simulink model "InverterGyro"  (R2020a)
settings: Solver=ode23tb  StartTime=0.0  StopTime=10.0  MaxStep=Tc
values from neighbouring files (symbols this model uses):
  cp = 40    [LD9_29rpm38.m]
  CTRPIFF_CLIP_RELEASE = 0.05    [InverterGyro_Init.m]
  emf_fb_p = 0.2*k    (= 0.4)    [LD9_29rpm38.m]
  emf_p = 0.08*k    (= 0.16)    [LD9_29rpm38.m]
  emf_valid = 0.25e3    (= 250)    [LD9_29rpm38.m]
  fcut_u_stack_flt = 161    [InverterGyro_Init.m]
  g0 = fcut_u_stack_flt * Tcontrol_INV    (= 0.0268333333333)    [InverterGyro_Init.m]
  g1 = 1 - g0    (= 0.973166666667)    [InverterGyro_Init.m]
  Ibez = In*sqrt(2)    [LD9_29rpm38.m]
  iq_lim = 1.4    [InverterGyro_Init.m]
  J = J    [plant_data.m]
  kalman_gamma = 1.6    [LD9_29rpm38.m]
  kalman_iq_est = 0    [LD9_29rpm38.m]
  kalman_w = kalman_gamma/k    (= 0.32)    [LD9_29rpm38.m]
  ki_inv_d = 18    [InverterGyro_Init.m]
  ki_inv_q = 18    [InverterGyro_Init.m]
  ki_w = 35    [InverterGyro_Init.m]
  kp_inv_d = 2    [InverterGyro_Init.m]
  kp_inv_q = 2    [InverterGyro_Init.m]
  kp_w = 8    [InverterGyro_Init.m]
  La = 1/3*(Lq+Ld)    (= 0.00188)    [LD9_29rpm38.m]
  Lb = 1/3*(Lq-Ld)    (= 0.00028)    [LD9_29rpm38.m]
  Ld_norm = Ld/Lbez    [LD9_29rpm38.m]
  LFi_0 = LFi_d/10    (= 8e-06)    [InverterGyro_Init.m]
  LFi_d = 80e-6    (= 8e-05)    [InverterGyro_Init.m]
  Ll = 5e-6    (= 5e-06)    [LD9_29rpm38.m]
  Lq_norm = Lq/Lbez    [LD9_29rpm38.m]
  Ls_norm = Ls/Lbez    [LD9_29rpm38.m]
  motorc_m_scale = 2/3*Vdc_nom/Ubez    [LD9_29rpm38.m]
  Omega_bez_motor = we_motor    (= 123.066656217)    [LD9_29rpm38.m]
  Omega_bez_plant = Omega_bez_motor * plant_motor_ratio    (= 123.066656217)    [LD9_29rpm38.m]
  Omega_bez_plant_m = Omega_bez_motor_m * plant_motor_ratio    (= 3.07666640542)    [LD9_29rpm38.m]
  phi = Ubez/Omega_bez_plant    [LD9_29rpm38.m]
  RLFi_0 = RLFi_d/3    (= 0.000334933333333)    [InverterGyro_Init.m]
  RLFi_d = 157*0.08*LFi_d    (= 0.0010048)    [InverterGyro_Init.m]
  Rs = 3.15e-3*n_modules    (= 0.0126)    [LD9_29rpm38.m]
  Rs_norm = Rs/Xbez    [LD9_29rpm38.m]
  settle_time = 0.1    [InverterGyro_Init.m]
  sign_speed = 1    [InverterGyro_Init.m]
  spdobs_emf_o_fact = 0    [LD9_29rpm38.m]
  spdobs_emf_q_fact = 0    [LD9_29rpm38.m]
  Tc = 1e-5    (= 1e-05)    [InverterGyro_Init.m]
  Tcontrol_INV = 1/fPWM_INV/2    (= 0.000166666666667)    [InverterGyro_Init.m]
  Tintcom = 100e-3    (= 0.1)    [InverterGyro_Init.m]
  Tload = 0.75*Tnom    (= 60750)    [LD9_29rpm38.m]
  Tnom = 324e3/n_modules    (= 81000)    [LD9_29rpm38.m]
  tref = 2    [InverterGyro_Init.m]
  Tsamp = Tc    (= 1e-05)    [InverterGyro_Init.m]
  udc_min = 0.85    [InverterGyro_Init.m]
  Vdc_nom = Vdc_ref    (= 720)    [InverterGyro_Init.m]    (also in LD9_29rpm38.m = Vdc_ref)
  Vdc_ref = 720    [InverterGyro_Init.m]
  wref = Omega_sim    [InverterGyro_Init.m]
undefined symbols (not defined in the file or in its folder): magnitude
libraries: powerlib x31, simulink x4, simulink_extras x4, cstblocks x1
(part 1 of 2)
settings Model: SimulationMode=accelerator  Creator=i0007573  LastModifiedBy=dbagn
settings SolverCC: ZeroCrossControl=EnableAll

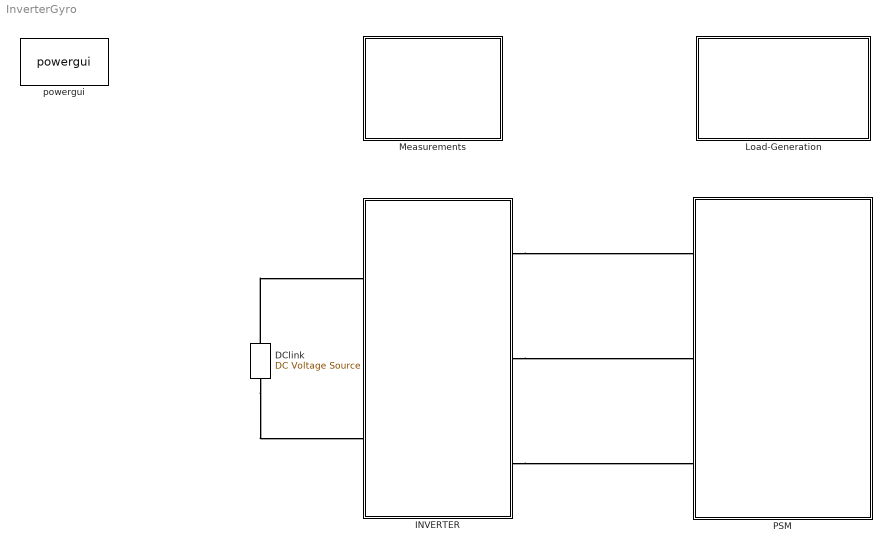
== system InverterGyro ==
  DClink : powerlib/Electrical Sources/DC Voltage Source  Amplitude=Vdc_ref  Measurements=None
  INVERTER : Subsystem
  Load-Generation : Subsystem
  Measurements : Subsystem
  PSM : Subsystem
  powergui : powerlib/powergui  SimulationMode=Continuous  SampleTime=Tc/10  frequency=60  Iterations=50  frequencyindice=0  Pbase=100e6  ErrMax=1e-4  UnitsV=kV  UnitsW=MW  buscounter=0  FunctionMessages=off  echomessages=off  EnableUseOfTLC=off  CurrentSourceSwitches=off  DisableSnubberDevices=off  DisableRonSwitches=off  DisableVfSwitches=off  DisplayEquations=on  AutomaticDiscreteSolvers=off  SolverType=Tustin  Interpol=off  ExternalGateDelay=off  methode=off  Ts=0  x0status=blocks  SPID=off  SwTol=0  HookPort=off  NonlinearTolerance=1e-4  nMaxIteration=100  ContinueOnMaxIteration=off  RestoreLinks=warning  ResistiveCurrentMeasurement=off  Frange=[0:2:500]  Ylog=off  Xlog=on  ShowGrid=off  save=off  variable=ZData  structure=0  ZoomFFT=on  StartTime=0.0  cycles=1  DisplayStyle=1  fundamental=60  FreqAxis=off  MaxFrequency=1000  frequencyindicesteady=1  RmsSteady=1  display=off
  connections:
  INVERTER/RConn1 -- PSM/LConn1
  INVERTER/RConn2 -- PSM/LConn2
  INVERTER/RConn3 -- PSM/LConn3
  DClink/RConn1 -- INVERTER/LConn1
  DClink/LConn1 -- INVERTER/LConn2

== system InverterGyro/INVERTER ==
  GYRO : Subsystem
  INVERTER Control : Subsystem
  LFi4 : powerlib/Elements/Series RLC Branch  LConnTagsString=__new0  RConnTagsString=__new0  BranchType=RL  Resistance=0  Inductance=1e-6  SetiL0=off  InitialCurrent=RLFi  Capacitance=1.0  Setx0=off  InitialVoltage=0  Measurements=Branch voltage and current
  LFi5 : powerlib/Elements/Series RLC Branch  LConnTagsString=__new0  RConnTagsString=__new0  BranchType=RL  Resistance=0  Inductance=1e-6  SetiL0=off  InitialCurrent=RLFi  Capacitance=1.0  Setx0=off  InitialVoltage=0  Measurements=Branch voltage and current
  LFi6 : powerlib/Elements/Series RLC Branch  LConnTagsString=__new0  RConnTagsString=__new0  BranchType=RL  Resistance=0  Inductance=1e-6  SetiL0=off  InitialCurrent=RLFi  Capacitance=1.0  Setx0=off  InitialVoltage=0  Measurements=Branch voltage and current
  LFi_INV1 : powerlib/Elements/Three-Phase Mutual Inductance Z1-Z0  LConnTagsString=a|b|c  RConnTagsString=A|B|C  PositiveSequence=[ RLFi_d LFi_d]  ZeroSequence=[ RLFi_0 LFi_0]
      settings: SourceProductBaseCode=PS
  V1in : PMIOPort  Side=Right
  V2in : PMIOPort  Port=2  Side=Right
  V3in : PMIOPort  Port=3  Side=Right
  DCbus+ : PMIOPort  Port=4  Side=Left
  DCbus- : PMIOPort  Port=5  Side=Left
  wires:
  INVERTER Control/1(PWMout) -> GYRO/1(m)
  connections:
  DCbus-/RConn1 -- GYRO/LConn2
  GYRO/LConn1 -- DCbus+/RConn1
  GYRO/RConn1 -- LFi4/LConn1
  LFi_INV1/RConn1 -- LFi4/RConn1
  LFi_INV1/RConn3 -- LFi6/RConn1
  GYRO/RConn3 -- LFi6/LConn1
  LFi_INV1/RConn2 -- LFi5/RConn1
  GYRO/RConn2 -- LFi5/LConn1
  LFi_INV1/LConn1 -- V1in/RConn1
  LFi_INV1/LConn2 -- V2in/RConn1
  LFi_INV1/LConn3 -- V3in/RConn1

== system InverterGyro/Load-Generation ==
  Gain1 : Gain
  Gain3 : Gain
  Saturation1 : Saturate  UpperLimit=Tload  LowerLimit=0
  To Workspace3 : ToWorkspace  VariableName=Tload_sim  SampleTime=Tc
      settings: MaxDataPoints=Nc
  Transfer Fcn : TransferFcn  Denominator=[1e-2 1]
  tload_ref : simulink/Sources/Ramp  slope=Tnom  start=start_torque_control  InitialOutput=0
  tag scope: Tload_applied=global
  wires:
  tload_ref/1 -> Saturation1/1
  Transfer Fcn/1 -> Gain3/1, To Workspace3/1
  Gain1/1 -> Transfer Fcn/1
  Saturation1/1 -> Gain1/1
  Gain3/1 -> [Tload_applied]

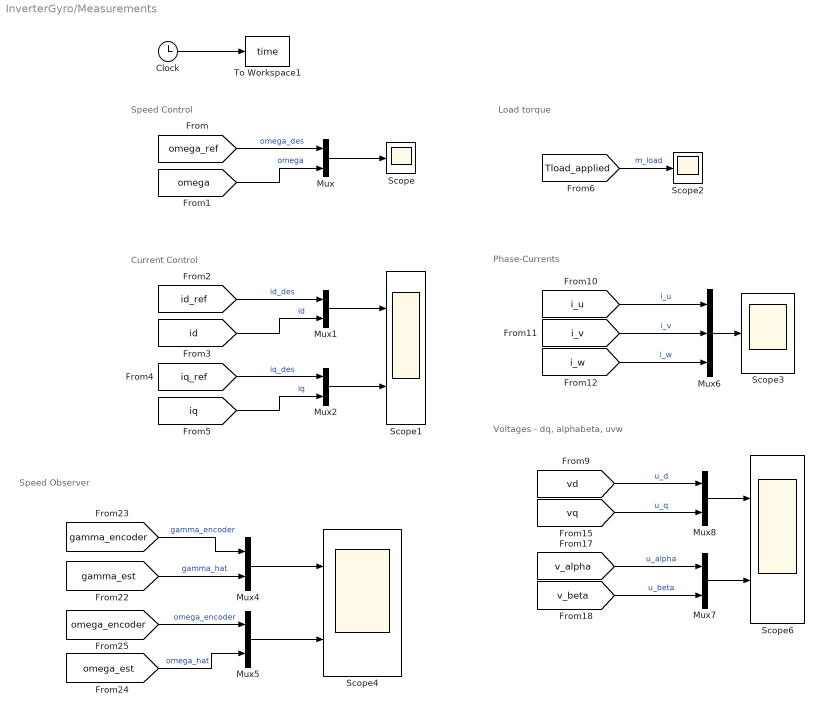
== system InverterGyro/Measurements ==
  note: Speed Observer
  note: Speed Control
  note: Current Control
  note: Load torque
  note: Phase-Currents
  note: Voltages - dq, alphabeta, uvw
  Clock : Clock
  Mux{,1..2,4..5,7..8} (7 alike) : Mux  Inputs=2
  Mux6 : Mux  Inputs=3
  Scope : Scope
  Scope1 : Scope  NumInputPorts=2
  Scope2 : Scope
  Scope3 : Scope
  Scope4 : Scope  NumInputPorts=2
  Scope6 : Scope  NumInputPorts=2
  To Workspace1 : ToWorkspace  VariableName=time  SampleTime=Tc
      settings: MaxDataPoints=Nc
  wires:
  Mux/1 -> Scope/1
  [omega_ref] -> Mux/1  "omega_des"
  [omega] -> Mux/2  "omega"
  Mux1/1 -> Scope1/1
  [id_ref] -> Mux1/1  "id_des"
  [id] -> Mux1/2  "id"
  [iq_ref] -> Mux2/1  "iq_des"
  [iq] -> Mux2/2  "iq"
  Mux2/1 -> Scope1/2
  Mux5/1 -> Scope4/2
  [gamma_encoder] -> Mux4/1  "gamma_encoder"
  Mux4/1 -> Scope4/1
  [omega_encoder] -> Mux5/1  "omega_encoder"
  [omega_est] -> Mux5/2  "omega_hat"
  [gamma_est] -> Mux4/2  "gamma_hat"
  [Tload_applied] -> Scope2/1  "m_load"
  Mux6/1 -> Scope3/1
  [i_u] -> Mux6/1  "i_u"
  [i_v] -> Mux6/2  "i_v"
  [i_w] -> Mux6/3  "i_w"
  [v_beta] -> Mux7/2  "u_beta"
  [v_alpha] -> Mux7/1  "u_alpha"
  [vd] -> Mux8/1  "u_d"
  [vq] -> Mux8/2  "u_q"
  Mux8/1 -> Scope6/1
  Mux7/1 -> Scope6/2
  Clock/1 -> To Workspace1/1

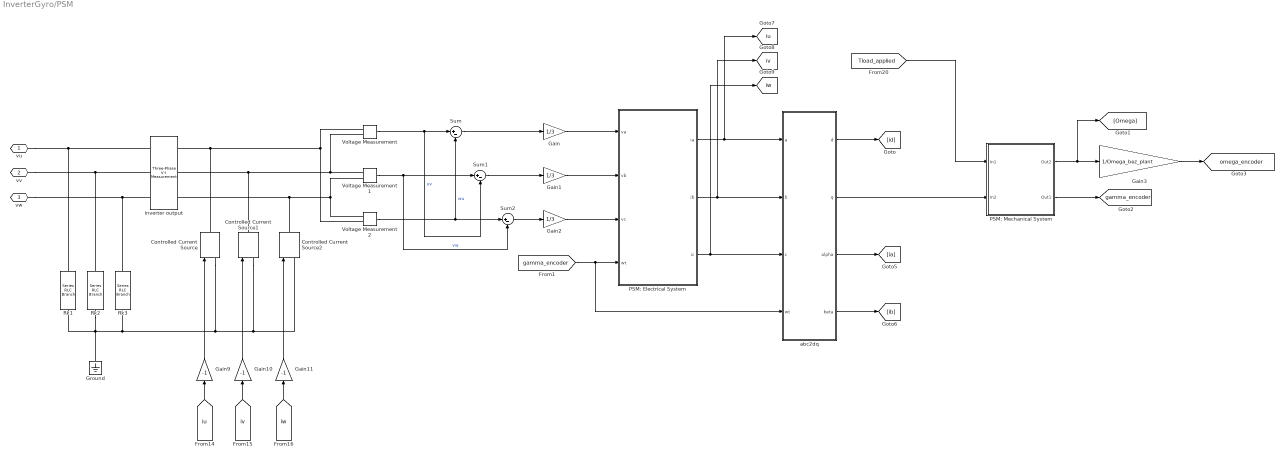
== system InverterGyro/PSM ==
  Controlled Current Source : powerlib/Electrical Sources/Controlled Current Source  Initialize=on  Source_Type=AC  Amplitude=0  Phase=0  Frequency=0  Measurements=None
  Controlled Current Source1 : powerlib/Electrical Sources/Controlled Current Source  Initialize=on  Source_Type=AC  Amplitude=0  Phase=0  Frequency=0  Measurements=None
  Controlled Current Source2 : powerlib/Electrical Sources/Controlled Current Source  Initialize=on  Source_Type=AC  Amplitude=0  Phase=0  Frequency=0  Measurements=None
  Gain : Gain  Gain=1/3
  Gain1 : Gain  Gain=1/3
  Gain10 : Gain  Gain=-1
  Gain11 : Gain  Gain=-1
  Gain2 : Gain  Gain=1/3
  Gain3 : Gain  Gain=1/Omega_bez_plant
  Gain9 : Gain  Gain=-1
  Ground : powerlib/Elements/Ground  LConnTagsString=a
  PSM: Electrical System : Subsystem
  PSM: Mechanical System : Subsystem
  Rk1 : powerlib/Elements/Series RLC Branch  LConnTagsString=__new0  RConnTagsString=__new0  BranchType=R  Resistance=1e6  Inductance=1e-3  SetiL0=off  InitialCurrent=0  Capacitance=1e-6  Setx0=off  InitialVoltage=0  Measurements=Branch voltage
  Rk2 : powerlib/Elements/Series RLC Branch  LConnTagsString=__new0  RConnTagsString=__new0  BranchType=R  Resistance=1e6  Inductance=1e-3  SetiL0=off  InitialCurrent=0  Capacitance=1e-6  Setx0=off  InitialVoltage=0  Measurements=Branch voltage
  Rk3 : powerlib/Elements/Series RLC Branch  LConnTagsString=__new0  RConnTagsString=__new0  BranchType=R  Resistance=1e6  Inductance=1e-3  SetiL0=off  InitialCurrent=0  Capacitance=1e-6  Setx0=off  InitialVoltage=0  Measurements=Branch voltage
  Sum : Sum  Inputs=|+-
  Sum1 : Sum  Inputs=|+-
  Sum2 : Sum  Inputs=|+-
  Voltage Measurement : powerlib/Measurements/Voltage Measurement  PhasorSimulation=off  OutputType=Complex  PSBequivalent=0
  Voltage Measurement1 : powerlib/Measurements/Voltage Measurement  PhasorSimulation=off  OutputType=Complex  PSBequivalent=0
  Voltage Measurement2 : powerlib/Measurements/Voltage Measurement  PhasorSimulation=off  OutputType=Complex  PSBequivalent=0
  "abc2dq " : Subsystem
  inverter output : powerlib/Measurements/Three-Phase V-I Measurement  VoltageMeasurement=phase-to-ground  SetLabelV=on  LabelV=Vgenerator1  Vpu=off  VpuLL=off  CurrentMeasurement=yes  SetLabelI=on  LabelI=Igenerator1  Ipu=off  Pbase=100e6  Vbase=500e3  OutputType=Complex  PhasorSimulation=off  PSBequivalent=0
  vu : PMIOPort  Side=Left
  vv : PMIOPort  Port=2  Side=Left
  vw : PMIOPort  Port=3  Side=Left
  tag scope: gamma_encoder=global, iu=global, iv=global, iw=global, omega_encoder=global
  wires:
  Sum2/1 -> Gain2/1
  Sum1/1 -> Gain1/1
  Sum/1 -> Gain/1
  Voltage Measurement2/1 -> Sum2/1, Sum/2  "wu"
  Voltage Measurement1/1 -> Sum2/2, Sum1/1  "vw"
  Voltage Measurement/1 -> Sum1/2, Sum/1  "uv"
  "abc2dq "/1(d) -> [id]
  [iu] -> Gain9/1
  [iv] -> Gain10/1
  [iw] -> Gain11/1
  Gain9/1 -> Controlled Current Source/1
  Gain10/1 -> Controlled Current Source1/1
  Gain11/1 -> Controlled Current Source2/1
  Gain/1 -> PSM: Electrical System/1(va)
  Gain1/1 -> PSM: Electrical System/2(vb)
  Gain2/1 -> PSM: Electrical System/3(vc)
  PSM: Electrical System/3(ic) -> [iw], "abc2dq "/3(c)
  PSM: Electrical System/2(ib) -> [iv], "abc2dq "/2(b)
  PSM: Electrical System/1(ia) -> [iu], "abc2dq "/1(a)
  "abc2dq "/3(alpha) -> [ia]
  "abc2dq "/4(beta) -> [ib]
  [Tload_applied] -> PSM: Mechanical System/1(In1)
  "abc2dq "/2(q) -> PSM: Mechanical System/2(In2)
  PSM: Mechanical System/1(Out2) -> Gain3/1, [Omega]
  PSM: Mechanical System/2(Out1) -> [gamma_encoder]
  [gamma_encoder] -> "abc2dq "/4(wt), PSM: Electrical System/4(wt)
  Gain3/1 -> [omega_encoder]
  connections:
  Voltage Measurement2/LConn1 -- Controlled Current Source2/RConn1 -- inverter output/RConn1 -- Voltage Measurement1/LConn2
  Voltage Measurement1/LConn1 -- Controlled Current Source1/RConn1 -- inverter output/RConn2 -- Voltage Measurement/LConn2
  Voltage Measurement/LConn1 -- Controlled Current Source/RConn1 -- inverter output/RConn3 -- Voltage Measurement2/LConn2
  Rk1/RConn1 -- Rk2/RConn1 -- Ground/LConn1 -- Controlled Current Source/LConn1 -- Controlled Current Source1/LConn1 -- Controlled Current Source2/LConn1 -- Rk3/RConn1
  Rk3/LConn1 -- vw/RConn1 -- inverter output/LConn1
  Rk2/LConn1 -- vv/RConn1 -- inverter output/LConn2
  Rk1/LConn1 -- vu/RConn1 -- inverter output/LConn3

== system InverterGyro/INVERTER/GYRO ==
  m : Inport
  Demux : Demux  Outputs=3
  Ground : powerlib/Elements/Ground  LConnTagsString=a
  gyro_one_phase : Subsystem
  gyro_one_phase1 : Subsystem
  gyro_one_phase2 : Subsystem
  A : PMIOPort  Side=Right
  B : PMIOPort  Port=2  Side=Right
  C : PMIOPort  Port=3  Side=Right
  V+ : PMIOPort  Port=4  Side=Left
  V- : PMIOPort  Port=5  Side=Left
  wires:
  Demux/1 -> gyro_one_phase/1(m)
  Demux/2 -> gyro_one_phase1/1(m)
  m/1 -> Demux/1
  Demux/3 -> gyro_one_phase2/1(m)
  connections:
  V+/RConn1 -- gyro_one_phase1/LConn1 -- gyro_one_phase2/LConn1 -- gyro_one_phase/LConn1
  V-/RConn1 -- gyro_one_phase/LConn2 -- gyro_one_phase1/LConn2 -- gyro_one_phase2/LConn2
  gyro_one_phase/RConn1 -- A/RConn1
  gyro_one_phase/RConn2 -- gyro_one_phase1/RConn2 -- Ground/LConn1 -- gyro_one_phase2/RConn2
  gyro_one_phase1/RConn1 -- B/RConn1
  gyro_one_phase2/RConn1 -- C/RConn1

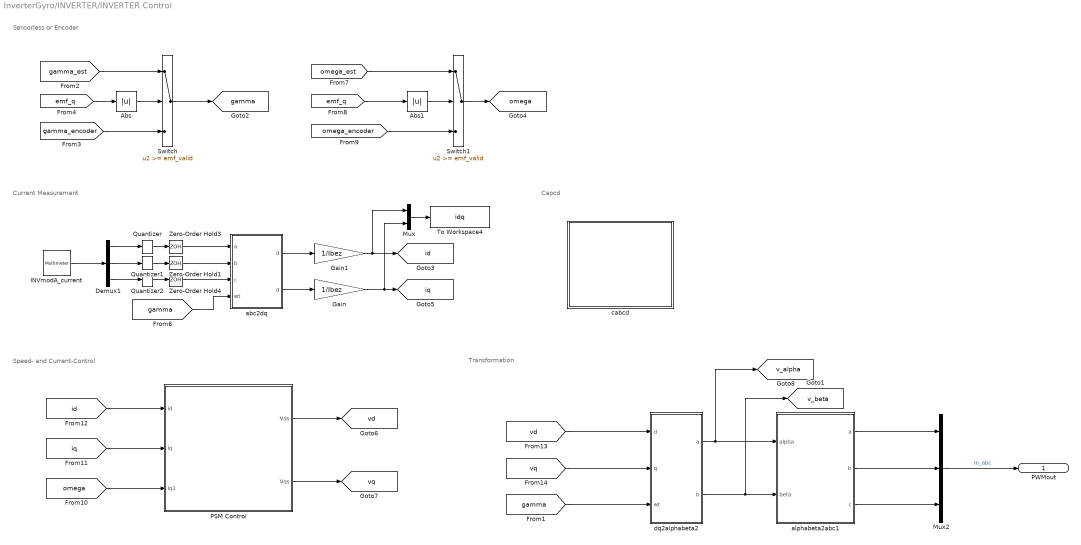
== system InverterGyro/INVERTER/INVERTER Control ==
  note: Capcd
  note: Transformation
  note: Speed- and Current-Control
  note: Current Measurement
  note: Sensorless or Encoder
  Abs : Abs
  Abs1 : Abs
  Demux1 : Demux  Outputs=3
  Gain : Gain  Gain=1/Ibez
  Gain1 : Gain  Gain=1/Ibez
  INVmodA_current : powerlib/Measurements/Multimeter  PhasorSimulation=off  OutputType=Complex  sel=[7 8 9]  L=9  Gain=[1 1 1]  yselected={'Ib: INVERTER/LFi4','Ib: INVERTER/LFi5','Ib: INVERTER/LFi6'};  PSBOutputType=1  PSBequivalent=0  AxesSetting=[0,0.1,-100,100]  Display=0  SavedBlockNames=-11
  Mux : Mux  Inputs=2
  Mux2 : Mux  Inputs=3
  PSM Control : Subsystem
  Quantizer : Quantizer  QuantizationInterval=CurrentQuantization
  Quantizer1 : Quantizer  QuantizationInterval=CurrentQuantization
  Quantizer2 : Quantizer  QuantizationInterval=CurrentQuantization
  Switch : Switch  Threshold=emf_valid
  Switch1 : Switch  Threshold=emf_valid
  To Workspace4 : ToWorkspace  VariableName=idq  SampleTime=Tc
      settings: MaxDataPoints=Nc
  Zero-Order Hold1 : ZeroOrderHold  SampleTime=Tcontrol_INV
  Zero-Order Hold3 : ZeroOrderHold  SampleTime=Tcontrol_INV
  Zero-Order Hold4 : ZeroOrderHold  SampleTime=Tcontrol_INV
  "abc2dq " : Subsystem
  alphabeta2abc1 : Subsystem
  cabcd : Subsystem
  dq2alphabeta2 : Subsystem
  PWMout : Outport
  tag scope: gamma=global, id=global, iq=global, omega=global, v_alpha=global, v_beta=global, vd=global, vq=global
  wires:
  Demux1/2 -> Quantizer1/1
  INVmodA_current/1 -> Demux1/1
  Demux1/3 -> Quantizer2/1
  "abc2dq "/1(d) -> Gain1/1
  "abc2dq "/2(q) -> Gain/1
  Zero-Order Hold3/1 -> "abc2dq "/1(a)
  Zero-Order Hold1/1 -> "abc2dq "/2(b)
  Zero-Order Hold4/1 -> "abc2dq "/3(c)
  Quantizer/1 -> Zero-Order Hold3/1
  Quantizer1/1 -> Zero-Order Hold1/1
  Quantizer2/1 -> Zero-Order Hold4/1
  [gamma_est] -> Switch/1
  [emf_q] -> Abs/1
  Abs/1 -> Switch/2
  Demux1/1 -> Quantizer/1
  [gamma] -> "abc2dq "/4(wt)
  Abs1/1 -> Switch1/2
  [emf_q] -> Abs1/1
  [omega_est] -> Switch1/1
  [omega_encoder] -> Switch1/3
  [omega] -> PSM Control/3(iq1)
  Gain1/1 -> Mux/1, [id]
  Gain/1 -> Mux/2, [iq]
  Mux/1 -> To Workspace4/1
  [id] -> PSM Control/1(id)
  [iq] -> PSM Control/2(iq)
  PSM Control/1(Vds) -> [vd]
  PSM Control/2(Vqs) -> [vq]
  [vd] -> dq2alphabeta2/1(d)
  [vq] -> dq2alphabeta2/2(q)
  [gamma_encoder] -> Switch/3
  Switch/1 -> [gamma]
  Switch1/1 -> [omega]
  dq2alphabeta2/1(a) -> [v_alpha], alphabeta2abc1/1(alpha)
  dq2alphabeta2/2(b) -> [v_beta], alphabeta2abc1/2(beta)
  alphabeta2abc1/1(a) -> Mux2/1
  alphabeta2abc1/2(b) -> Mux2/2
  alphabeta2abc1/3(c) -> Mux2/3
  Mux2/1 -> PWMout/1  "m_abc"
  [gamma] -> dq2alphabeta2/3(wt)

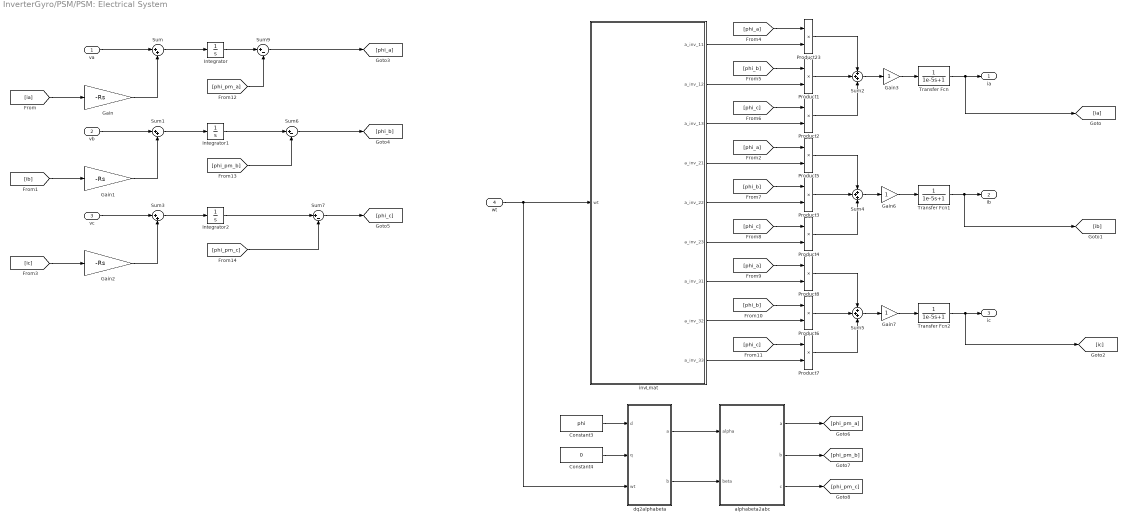
== system InverterGyro/PSM/PSM: Electrical System ==
  va : Inport
  vb : Inport  Port=2
  vc : Inport  Port=3
  wt : Inport  Port=4
  Constant3 : Constant  Value=phi
  Constant4 : Constant  Value=0
  Gain : Gain  Gain=-Rs
  Gain1 : Gain  Gain=-Rs
  Gain2 : Gain  Gain=-Rs
  Gain3 : Gain
  Gain6 : Gain
  Gain7 : Gain
  Integrator : Integrator  InitialCondition=phi
  Integrator1 : Integrator  InitialCondition=phi*cos(2*pi/3)
  Integrator2 : Integrator  InitialCondition=phi*cos(-2*pi/3)
  Product{1..8,23} (9 alike) : Product
  Sum : Sum  Inputs=|++
  Sum1 : Sum  Inputs=|++
  Sum2 : Sum  Inputs=+++
  Sum3 : Sum  Inputs=|++
  Sum4 : Sum  Inputs=+++
  Sum5 : Sum  Inputs=+++
  Sum6 : Sum  Inputs=|+-
  Sum7 : Sum  Inputs=|+-
  Sum9 : Sum  Inputs=|+-
  Transfer Fcn : TransferFcn  Denominator=[1e-5 1]
  Transfer Fcn1 : TransferFcn  Denominator=[1e-5 1]
  Transfer Fcn2 : TransferFcn  Denominator=[1e-5 1]
  alphabeta2abc : Subsystem
  dq2alphabeta : Subsystem
  invLmat : Subsystem
  ia : Outport
  ib : Outport  Port=2
  ic : Outport  Port=3
  wires:
  va/1 -> Sum/1
  Gain/1 -> Sum/2
  [ia] -> Gain/1
  Sum/1 -> Integrator/1
  vb/1 -> Sum1/1
  Gain1/1 -> Sum1/2
  Sum1/1 -> Integrator1/1
  [ib] -> Gain1/1
  vc/1 -> Sum3/1
  Gain2/1 -> Sum3/2
  [ic] -> Gain2/1
  Sum3/1 -> Integrator2/1
  wt/1 -> invLmat/1(wt), dq2alphabeta/3(wt)
  [phi_a] -> Product23/1
  invLmat/1(a_inv_11) -> Product23/2
  [phi_b] -> Product1/1
  invLmat/2(a_inv_12) -> Product1/2
  [phi_c] -> Product2/1
  invLmat/3(a_inv_13) -> Product2/2
  [phi_a] -> Product5/1
  invLmat/4(a_inv_21) -> Product5/2
  [phi_b] -> Product3/1
  invLmat/5(a_inv_22) -> Product3/2
  [phi_c] -> Product4/1
  invLmat/6(a_inv_23) -> Product4/2
  [phi_a] -> Product8/1
  invLmat/7(a_inv_31) -> Product8/2
  [phi_b] -> Product6/1
  invLmat/8(a_inv_32) -> Product6/2
  [phi_c] -> Product7/1
  invLmat/9(a_inv_33) -> Product7/2
  Product1/1 -> Sum2/2
  Product23/1 -> Sum2/1
  Product2/1 -> Sum2/3
  Product3/1 -> Sum4/2
  Product5/1 -> Sum4/1
  Product4/1 -> Sum4/3
  Product6/1 -> Sum5/2
  Product8/1 -> Sum5/1
  Product7/1 -> Sum5/3
  Transfer Fcn2/1 -> [ic], ic/1
  Transfer Fcn1/1 -> [ib], ib/1
  Transfer Fcn/1 -> [ia], ia/1
  Gain7/1 -> Transfer Fcn2/1
  Sum2/1 -> Gain3/1
  Sum4/1 -> Gain6/1
  Sum5/1 -> Gain7/1
  Constant3/1 -> dq2alphabeta/1(d)
  Constant4/1 -> dq2alphabeta/2(q)
  dq2alphabeta/1(a) -> alphabeta2abc/1(alpha)
  dq2alphabeta/2(b) -> alphabeta2abc/2(beta)
  Gain3/1 -> Transfer Fcn/1
  Gain6/1 -> Transfer Fcn1/1
  Integrator/1 -> Sum9/1
  Integrator1/1 -> Sum6/1
  Sum6/1 -> [phi_b]
  Sum7/1 -> [phi_c]
  Integrator2/1 -> Sum7/1
  alphabeta2abc/1(a) -> [phi_pm_a]
  alphabeta2abc/2(b) -> [phi_pm_b]
  alphabeta2abc/3(c) -> [phi_pm_c]
  Sum9/1 -> [phi_a]
  [phi_pm_a] -> Sum9/2
  [phi_pm_b] -> Sum6/2
  [phi_pm_c] -> Sum7/2

== system InverterGyro/PSM/PSM: Mechanical System ==
  In1 : Inport
  In2 : Inport  Port=2
  Constant : Constant  Value=phi
  Constant2 : Constant  Value=2*pi
  Gain5 : Gain  Gain=cp
  Gain6 : Gain  Gain=cp
  Gain8 : Gain  Gain=3/2
  Integrator : Integrator
  Integrator1 : Integrator
  Math Function2 : Math  Operator=mod  SignedPower=on  SaturateOnIntegerOverflow=on
  Product : Product
  Product1 : Product
  Sum5 : Sum  Inputs=|+-
  plant_inertia : Subsystem
  Out2 : Outport
  Out1 : Outport  Port=2
  wires:
  Integrator/1 -> Gain6/1
  Gain6/1 -> Integrator1/1, Out2/1, [Omega]  "Omega"
  plant_inertia/1(J_1) -> Product1/2
  In2/1 -> [iq], Product/1  "iq"
  Integrator1/1 -> Math Function2/1  "wt"
  Constant/1 -> Product/2
  Gain8/1 -> [Te], Sum5/1
  Constant2/1 -> Math Function2/2
  Gain5/1 -> Gain8/1
  Sum5/1 -> Product1/1
  Product/1 -> Gain5/1
  Math Function2/1 -> Out1/1, [theta_m]  "gamma"
  Product1/1 -> Integrator/1
  In1/1 -> Sum5/2  "m_load"

== system InverterGyro/PSM/abc2dq  ==
  a : Inport
  b : Inport  Port=2
  c : Inport  Port=3
  wt : Inport  Port=4
  abc2alphabeta : Subsystem
  alphabeta2dq : Subsystem
  d : Outport
  q : Outport  Port=2
  alpha : Outport  Port=3
  beta : Outport  Port=4
  wires:
  c/1 -> abc2alphabeta/3(c)
  b/1 -> abc2alphabeta/2(b)
  a/1 -> abc2alphabeta/1(a)
  abc2alphabeta/1("alpha ") -> alpha/1, alphabeta2dq/1(alpha)
  abc2alphabeta/2("beta ") -> beta/1, alphabeta2dq/2(beta)
  wt/1 -> alphabeta2dq/3(wt)
  alphabeta2dq/1(d) -> d/1
  alphabeta2dq/2(q) -> q/1

== system InverterGyro/INVERTER/GYRO/gyro_one_phase ==
  m : Inport
  Controlled Current Source2 : powerlib/Electrical Sources/Controlled Current Source  Initialize=on  Source_Type=AC  Amplitude=0  Phase=0  Frequency=0  Measurements=None
  Controlled Voltage Source : powerlib/Electrical Sources/Controlled Voltage Source  Initialize=on  Source_Type=AC  Amplitude=0  Phase=0  Frequency=0  Measurements=None
  Current Measurement : powerlib/Measurements/Current Measurement  PhasorSimulation=off  OutputType=Complex  PSBequivalent=0
  Product : Product
  Product1 : Product
  Transfer Fcn1 : TransferFcn  Denominator=[1e-4 1]
  Transfer Fcn2 : TransferFcn  Denominator=[1e-4 1]
  Voltage Measurement : powerlib/Measurements/Voltage Measurement  PhasorSimulation=off  OutputType=Complex  PSBequivalent=0
  A : PMIOPort  Side=Left
  B : PMIOPort  Port=2  Side=Left
  a : PMIOPort  Port=3  Side=Right
  b : PMIOPort  Port=4  Side=Right
  wires:
  m/1 -> Product1/2, Product/2
  Product/1 -> Controlled Voltage Source/1
  Voltage Measurement/1 -> Transfer Fcn2/1
  Product1/1 -> Controlled Current Source2/1
  Current Measurement/1 -> Transfer Fcn1/1
  Transfer Fcn2/1 -> Product/1
  Transfer Fcn1/1 -> Product1/1
  connections:
  A/RConn1 -- Voltage Measurement/LConn1 -- Controlled Current Source2/LConn1
  Controlled Current Source2/RConn1 -- B/RConn1 -- Voltage Measurement/LConn2
  Controlled Voltage Source/LConn1 -- b/RConn1
  Controlled Voltage Source/RConn1 -- Current Measurement/LConn1
  Current Measurement/RConn1 -- a/RConn1

== system InverterGyro/INVERTER/GYRO/gyro_one_phase1 ==
  m : Inport
  Controlled Current Source2 : powerlib/Electrical Sources/Controlled Current Source  Initialize=on  Source_Type=AC  Amplitude=0  Phase=0  Frequency=0  Measurements=None
  Controlled Voltage Source : powerlib/Electrical Sources/Controlled Voltage Source  Initialize=on  Source_Type=AC  Amplitude=0  Phase=0  Frequency=0  Measurements=None
  Current Measurement : powerlib/Measurements/Current Measurement  PhasorSimulation=off  OutputType=Complex  PSBequivalent=0
  Product : Product
  Product1 : Product
  Transfer Fcn1 : TransferFcn  Denominator=[1e-4 1]
  Transfer Fcn2 : TransferFcn  Denominator=[1e-4 1]
  Voltage Measurement : powerlib/Measurements/Voltage Measurement  PhasorSimulation=off  OutputType=Complex  PSBequivalent=0
  A : PMIOPort  Side=Left
  B : PMIOPort  Port=2  Side=Left
  a : PMIOPort  Port=3  Side=Right
  b : PMIOPort  Port=4  Side=Right
  wires:
  m/1 -> Product1/2, Product/2
  Product/1 -> Controlled Voltage Source/1
  Voltage Measurement/1 -> Transfer Fcn2/1
  Product1/1 -> Controlled Current Source2/1
  Current Measurement/1 -> Transfer Fcn1/1
  Transfer Fcn2/1 -> Product/1
  Transfer Fcn1/1 -> Product1/1
  connections:
  A/RConn1 -- Voltage Measurement/LConn1 -- Controlled Current Source2/LConn1
  Controlled Current Source2/RConn1 -- B/RConn1 -- Voltage Measurement/LConn2
  Controlled Voltage Source/LConn1 -- b/RConn1
  Controlled Voltage Source/RConn1 -- Current Measurement/LConn1
  Current Measurement/RConn1 -- a/RConn1

== system InverterGyro/INVERTER/GYRO/gyro_one_phase2 ==
  m : Inport
  Controlled Current Source2 : powerlib/Electrical Sources/Controlled Current Source  Initialize=on  Source_Type=AC  Amplitude=0  Phase=0  Frequency=0  Measurements=None
  Controlled Voltage Source : powerlib/Electrical Sources/Controlled Voltage Source  Initialize=on  Source_Type=AC  Amplitude=0  Phase=0  Frequency=0  Measurements=None
  Current Measurement : powerlib/Measurements/Current Measurement  PhasorSimulation=off  OutputType=Complex  PSBequivalent=0
  Product : Product
  Product1 : Product
  Transfer Fcn1 : TransferFcn  Denominator=[1e-4 1]
  Transfer Fcn2 : TransferFcn  Denominator=[1e-4 1]
  Voltage Measurement : powerlib/Measurements/Voltage Measurement  PhasorSimulation=off  OutputType=Complex  PSBequivalent=0
  A : PMIOPort  Side=Left
  B : PMIOPort  Port=2  Side=Left
  a : PMIOPort  Port=3  Side=Right
  b : PMIOPort  Port=4  Side=Right
  wires:
  m/1 -> Product1/2, Product/2
  Product/1 -> Controlled Voltage Source/1
  Voltage Measurement/1 -> Transfer Fcn2/1
  Product1/1 -> Controlled Current Source2/1
  Current Measurement/1 -> Transfer Fcn1/1
  Transfer Fcn2/1 -> Product/1
  Transfer Fcn1/1 -> Product1/1
  connections:
  A/RConn1 -- Voltage Measurement/LConn1 -- Controlled Current Source2/LConn1
  Controlled Current Source2/RConn1 -- B/RConn1 -- Voltage Measurement/LConn2
  Controlled Voltage Source/LConn1 -- b/RConn1
  Controlled Voltage Source/RConn1 -- Current Measurement/LConn1
  Current Measurement/RConn1 -- a/RConn1

== system InverterGyro/INVERTER/INVERTER Control/PSM Control ==
  note: EMF & Luenberger Observer
  note: Current Control
  note: Speed Control
  id : Inport
  iq : Inport  Port=2
  iq1 : Inport  Port=3
  Current control : Subsystem
  References : Subsystem
  Speed control : Subsystem
  observer : Subsystem
  speed reference : Subsystem
  Vds : Outport
  Vqs : Outport  Port=2
  tag scope: T_ref=global, gamma_est=global, iq_est=global, omega_est=global
  wires:
  References/1(Id_ref) -> Current control/1(Id_ref)
  References/2(Iq_ref) -> Current control/2(Iq_ref)
  Current control/1(vd) -> Vds/1  "vd"
  Current control/2(vq) -> Vqs/1  "vq"
  speed reference/1(ref_out) -> Speed control/2(Speed ref)
  [i_alpha] -> observer/1(ia_s)
  [i_beta] -> observer/2(ib_s)
  Speed control/1(Torque ref) -> [T_ref]
  [v_alpha] -> observer/3(va_s)
  [v_beta] -> observer/4(vb_s)
  observer/3(iq_hat) -> [iq_est]
  iq1/1 -> Speed control/1(Rotor speed), Current control/3(omega)  "omega"
  id/1 -> Current control/4(id)  "id"
  iq/1 -> Current control/5(iq)  "iq"
  observer/1(iq_hat2) -> [omega_est]
  observer/2(iq_hat1) -> [gamma_est]

== system InverterGyro/INVERTER/INVERTER Control/abc2dq  ==
  a : Inport
  b : Inport  Port=2
  c : Inport  Port=3
  wt : Inport  Port=4
  1/Ti1 : Gain  Gain=1/Ibez  SaturateOnIntegerOverflow=on  OutDataTypeStr=Inherit: Same as input  ParamDataTypeStr=Inherit: Same as input
  1/Ti2 : Gain  Gain=1/Ibez  SaturateOnIntegerOverflow=on  OutDataTypeStr=Inherit: Same as input  ParamDataTypeStr=Inherit: Same as input
  To Workspace1 : ToWorkspace  VariableName=ib  SampleTime=Tc
      settings: MaxDataPoints=Nc
  To Workspace2 : ToWorkspace  VariableName=iq  SampleTime=Tc
      settings: MaxDataPoints=Nc
  To Workspace3 : ToWorkspace  VariableName=id  SampleTime=Tc
      settings: MaxDataPoints=Nc
  To Workspace4 : ToWorkspace  VariableName=ia  SampleTime=Tc
      settings: MaxDataPoints=Nc
  abc2alphabeta : Subsystem
  alphabeta2dq : Subsystem
  d : Outport
  q : Outport  Port=2
  tag scope: i_alpha=global, i_beta=global, i_u=global, i_v=global, i_w=global
  wires:
  wt/1 -> alphabeta2dq/3(wt)  "gamma"
  abc2alphabeta/2("beta ") -> To Workspace1/1, 1/Ti1/1, alphabeta2dq/2(beta)
  abc2alphabeta/1("alpha ") -> 1/Ti2/1, To Workspace4/1, alphabeta2dq/1(alpha)
  a/1 -> [i_u], abc2alphabeta/1(a)
  b/1 -> [i_v], abc2alphabeta/2(b)
  c/1 -> [i_w], abc2alphabeta/3(c)
  1/Ti2/1 -> [i_alpha]
  1/Ti1/1 -> [i_beta]
  alphabeta2dq/2(q) -> To Workspace2/1, q/1
  alphabeta2dq/1(d) -> To Workspace3/1, d/1

== system InverterGyro/INVERTER/INVERTER Control/alphabeta2abc1 ==
  alpha : Inport
  beta : Inport  Port=2
  Gain1 : Gain  Gain=0
  Gain2 : Gain  Gain=sqrt(3)/2
  Gain3 : Gain  Gain=-1/2
  Gain4 : Gain  Gain=-sqrt(3)/2
  Gain5 : Gain
  Gain6 : Gain  Gain=-1/2
  Sum : Sum
  Sum1 : Sum
  Sum2 : Sum
  a : Outport
  b : Outport  Port=2
  c : Outport  Port=3
  wires:
  Sum/1 -> a/1
  Sum1/1 -> b/1
  alpha/1 -> Gain6/1, Gain3/1, Gain5/1
  beta/1 -> Gain4/1, Gain2/1, Gain1/1
  Gain5/1 -> Sum/1
  Gain1/1 -> Sum/2
  Gain3/1 -> Sum1/1
  Gain2/1 -> Sum1/2
  Gain6/1 -> Sum2/1
  Gain4/1 -> Sum2/2
  Sum2/1 -> c/1

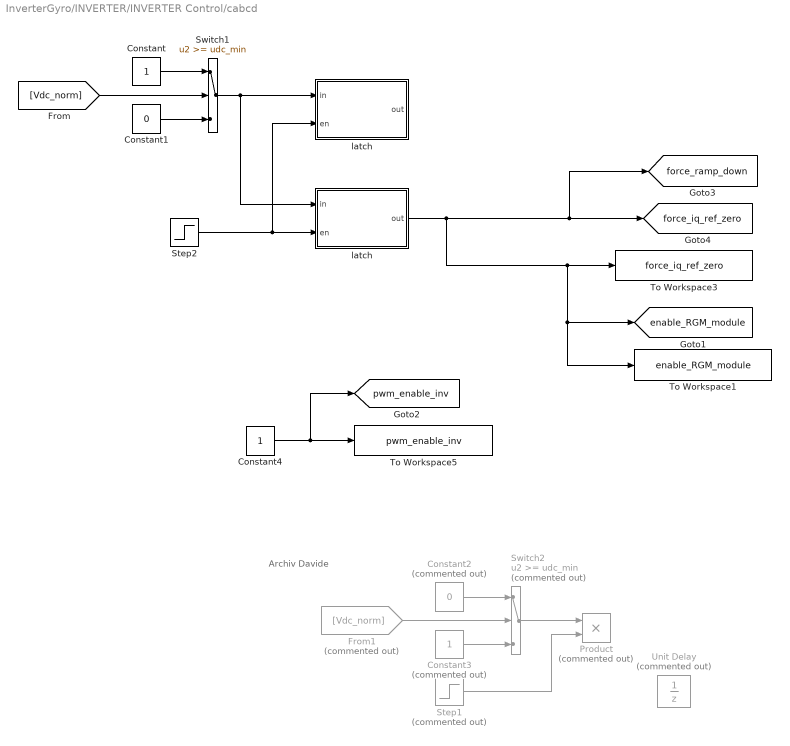
== system InverterGyro/INVERTER/INVERTER Control/cabcd ==
  note: Archiv Davide
  Constant : Constant
  Constant1 : Constant  Value=0
  Constant2 : Constant  Commented=on  Value=0
  Constant3 : Constant  Commented=on
  Constant4 : Constant
  From1 : From  Commented=on  GotoTag=Vdc_norm  TagVisibility=global
  Product : Product  Commented=on
  Step1 : Step  Commented=on  Time=settle_time  SampleTime=0
  Step2 : Step  Time=settle_time  SampleTime=0
  Switch1 : Switch  Threshold=udc_min
  Switch2 : Switch  Commented=on  Threshold=udc_min
  To Workspace1 : ToWorkspace  VariableName=enable_RGM_module  SampleTime=Tc
      settings: MaxDataPoints=Nc
  To Workspace3 : ToWorkspace  VariableName=force_iq_ref_zero  SampleTime=Tc
      settings: MaxDataPoints=Nc
  To Workspace5 : ToWorkspace  VariableName=pwm_enable_inv  SampleTime=Tc
      settings: MaxDataPoints=Nc
  Unit Delay : UnitDelay  Commented=on  SampleTime=Tintcom  HasFrameUpgradeWarning=on
  latch : Subsystem
  "latch " : Subsystem
  tag scope: enable_RGM_module=global, force_iq_ref_zero=global, force_ramp_down=global, pwm_enable_inv=global
  wires:
  Constant1/1 -> Switch1/3
  Constant/1 -> Switch1/1
  [Vdc_norm] -> Switch1/2
  Switch1/1 -> "latch "/1(in), latch/1(in)
  Constant3/1 -> Switch2/3
  Constant2/1 -> Switch2/1
  From1/1 -> Switch2/2
  Constant4/1 -> To Workspace5/1, [pwm_enable_inv]
  "latch "/1(out) -> [force_ramp_down], [force_iq_ref_zero], To Workspace1/1, [enable_RGM_module], To Workspace3/1
  Switch2/1 -> Product/1
  Step1/1 -> Product/2
  Step2/1 -> latch/2(en), "latch "/2(en)

== system InverterGyro/INVERTER/INVERTER Control/dq2alphabeta2 ==
  d : Inport
  q : Inport  Port=2
  wt : Inport  Port=3
  dq-alphabeta : Subsystem
  a : Outport
  b : Outport  Port=2
  wires:
  d/1 -> dq-alphabeta/1(d)
  q/1 -> dq-alphabeta/2(q)
  dq-alphabeta/1(alpha) -> a/1
  dq-alphabeta/2(beta) -> b/1
  wt/1 -> dq-alphabeta/3(wt)

== system InverterGyro/PSM/PSM: Electrical System/alphabeta2abc ==
  alpha : Inport
  beta : Inport  Port=2
  Gain1 : Gain  Gain=0
  Gain2 : Gain  Gain=sqrt(3)/2
  Gain3 : Gain  Gain=-1/2
  Gain4 : Gain  Gain=-sqrt(3)/2
  Gain5 : Gain
  Gain6 : Gain  Gain=-1/2
  Sum : Sum
  Sum1 : Sum
  Sum2 : Sum
  a : Outport
  b : Outport  Port=2
  c : Outport  Port=3
  wires:
  Sum/1 -> a/1
  Sum1/1 -> b/1
  alpha/1 -> Gain6/1, Gain3/1, Gain5/1
  beta/1 -> Gain4/1, Gain2/1, Gain1/1
  Gain5/1 -> Sum/1
  Gain1/1 -> Sum/2
  Gain3/1 -> Sum1/1
  Gain2/1 -> Sum1/2
  Gain6/1 -> Sum2/1
  Gain4/1 -> Sum2/2
  Sum2/1 -> c/1

== system InverterGyro/PSM/PSM: Electrical System/dq2alphabeta ==
  d : Inport
  q : Inport  Port=2
  wt : Inport  Port=3
  dq-alphabeta : Subsystem
  a : Outport
  b : Outport  Port=2
  wires:
  wt/1 -> dq-alphabeta/3(wt)
  dq-alphabeta/2(beta) -> b/1
  dq-alphabeta/1(alpha) -> a/1
  q/1 -> dq-alphabeta/2(q)
  d/1 -> dq-alphabeta/1(d)

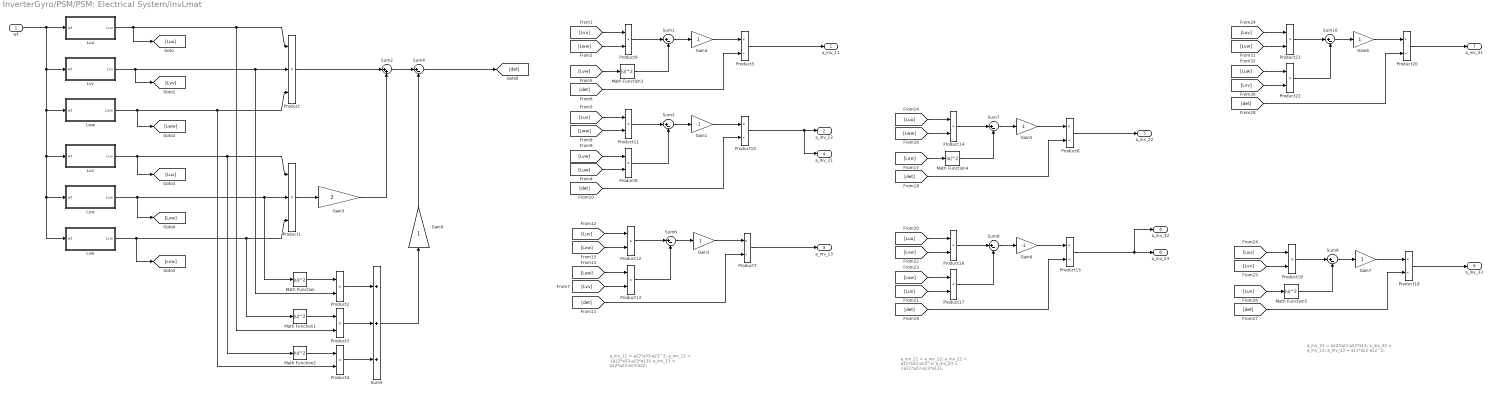
== system InverterGyro/PSM/PSM: Electrical System/invLmat ==
  note: a_inv_21 = a_inv_12;
      | a_inv_22 = a11*a33-a13^2;
      | a_inv_23 = -(a11*a23-a13*a12);
  note: a_inv_11 = a22*a33-a23^2;
      | a_inv_12 = -(a12*a33-a23*a13);
      | a_inv_13 = a12*a23-a13*a22;
  note: a_inv_31 = a12*a23-a22*a13;
      | a_inv_32 = a_inv_23;
      | a_inv_33 = a11*a22-a12^2;
  wt : Inport
  Gain1 : Gain  Gain=-1
  Gain{2,4..5,7..9} (6 alike) : Gain
  Gain3 : Gain  Gain=2
  Gain6 : Gain  Gain=-1
  Luu : Subsystem
  Luv : Subsystem
  Luw : Subsystem
  Lvv : Subsystem
  Lvw : Subsystem
  Lww : Subsystem
  Math Function{,1..5} (6 alike) : Math  Operator=magnitude^2  SignedPower=on  SaturateOnIntegerOverflow=on
  Product : Product  Inputs=3
  Product1 : Product  Inputs=3
  Product{5,7..8,10,15,18,20} (7 alike) : Product  Inputs=*/
  Product{2..4,6,9,11..14,16..17,19,21..22} (14 alike) : Product
  Sum{1,3..4,6..10} (8 alike) : Sum  Inputs=|+-
  Sum2 : Sum  Inputs=|++
  Sum5 : Sum  Inputs=+++
  a_inv_11 : Outport
  a_inv_12 : Outport  Port=2
  a_inv_13 : Outport  Port=3
  a_inv_21 : Outport  Port=4
  a_inv_22 : Outport  Port=5
  a_inv_23 : Outport  Port=6
  a_inv_31 : Outport  Port=7
  a_inv_32 : Outport  Port=8
  a_inv_33 : Outport  Port=9
  wires:
  Luw/1(Luw) -> [Luw], Math Function/1, Product1/2
  Product/1 -> Sum2/1
  wt/1 -> Lvw/1(wt), Luw/1(wt), Luv/1(wt), Lww/1(wt), Lvv/1(wt), Luu/1(wt)
  Lvv/1(Lvv) -> [Lvv], Product2/2, Product/2
  Math Function2/1 -> Product4/1
  Luu/1(Luu) -> Product3/2, Product/1, [Luu]
  Sum2/1 -> Sum4/1
  Lvw/1(Lvw) -> [Lvw], Math Function1/1, Product1/3
  Product4/1 -> Sum5/3
  Product3/1 -> Sum5/2
  Luv/1(Luv) -> [Luv], Math Function2/1, Product1/1
  Math Function1/1 -> Product3/1
  Lww/1(Lww) -> [Lww], Product4/2, Product/3
  Gain3/1 -> Sum2/2
  Product1/1 -> Gain3/1
  Math Function/1 -> Product2/1
  Product2/1 -> Sum5/1
  [Lww] -> Product9/2
  [Lvv] -> Product9/1
  Product9/1 -> Sum1/1
  Math Function3/1 -> Sum1/2
  [Lvw] -> Math Function3/1
  Sum1/1 -> Gain4/1
  [det] -> Product5/2
  Product11/1 -> Sum3/1
  Product6/1 -> Sum3/2
  Sum3/1 -> Gain1/1
  [det] -> Product10/2
  Gain1/1 -> Product10/1
  [Luv] -> Product11/1
  [Lww] -> Product11/2
  [Lvw] -> Product6/1
  [Luw] -> Product6/2
  Product12/1 -> Sum6/1
  Product13/1 -> Sum6/2
  Sum6/1 -> Gain2/1
  [det] -> Product7/2
  Gain2/1 -> Product7/1
  Gain4/1 -> Product5/1
  [Luv] -> Product12/1
  [Lvw] -> Product12/2
  [Luw] -> Product13/1
  [Lvv] -> Product13/2
  [Lww] -> Product14/2
  [Luu] -> Product14/1
  Product14/1 -> Sum7/1
  Math Function4/1 -> Sum7/2
  [Luw] -> Math Function4/1
  Sum7/1 -> Gain5/1
  [det] -> Product8/2
  Gain5/1 -> Product8/1
  Product16/1 -> Sum8/1
  Product17/1 -> Sum8/2
  Sum8/1 -> Gain6/1
  [det] -> Product15/2
  Gain6/1 -> Product15/1
  [Luu] -> Product16/1
  [Lvw] -> Product16/2
  [Luw] -> Product17/1
  [Luv] -> Product17/2
  [Lvv] -> Product19/2
  [Luu] -> Product19/1
  Product19/1 -> Sum9/1
  Math Function5/1 -> Sum9/2
  [Luv] -> Math Function5/1
  Sum9/1 -> Gain7/1
  [det] -> Product18/2
  Gain7/1 -> Product18/1
  Product21/1 -> Sum10/1
  Product22/1 -> Sum10/2
  Sum10/1 -> Gain8/1
  [det] -> Product20/2
  Gain8/1 -> Product20/1
  [Luv] -> Product21/1
  [Lvw] -> Product21/2
  [Luw] -> Product22/1
  [Lvv] -> Product22/2
  Sum4/1 -> [det]
  Sum5/1 -> Gain9/1
  Gain9/1 -> Sum4/2
  Product5/1 -> a_inv_11/1
  Product10/1 -> a_inv_21/1, a_inv_12/1
  Product7/1 -> a_inv_13/1
  Product8/1 -> a_inv_22/1
  Product15/1 -> a_inv_32/1, a_inv_23/1
  Product20/1 -> a_inv_31/1
  Product18/1 -> a_inv_33/1

== system InverterGyro/PSM/PSM: Mechanical System/plant_inertia ==
  Constant1 : Constant  Value=J
  Constant4 : Constant
  Product5 : Product  Inputs=*/
  To Workspace1 : ToWorkspace  VariableName=plant_inertia  SampleTime=Tc
      settings: MaxDataPoints=Nc
  J_1 : Outport
  wires:
  Product5/1 -> J_1/1
  Constant1/1 -> Product5/2, To Workspace1/1
  Constant4/1 -> Product5/1

== system InverterGyro/PSM/abc2dq /abc2alphabeta ==
  a : Inport
  b : Inport  Port=2
  c : Inport  Port=3
  Gain1 : Gain  Gain=-1/2
  Gain11 : Gain  Gain=-1/2
  Gain2 : Gain  Gain=0
  Gain3 : Gain  Gain=sqrt(3)/2
  Gain4 : Gain  Gain=-sqrt(3)/2
  Gain8 : Gain  Gain=2/3
  Gain9 : Gain  Gain=2/3
  Sum : Sum  Inputs=+++
  Sum1 : Sum  Inputs=+++
  "alpha " : Outport
  "beta " : Outport  Port=2
  wires:
  Gain9/1 -> "beta "/1
  Gain8/1 -> "alpha "/1
  Gain11/1 -> Sum/2
  Gain1/1 -> Sum/3
  Gain2/1 -> Sum1/1
  Gain3/1 -> Sum1/2
  Gain4/1 -> Sum1/3
  a/1 -> Gain2/1, Sum/1
  c/1 -> Gain4/1, Gain1/1
  b/1 -> Gain3/1, Gain11/1
  Sum/1 -> Gain8/1
  Sum1/1 -> Gain9/1

== system InverterGyro/PSM/abc2dq /alphabeta2dq ==
  alpha : Inport
  beta : Inport  Port=2
  wt : Inport  Port=3
  Product{,1..3} (4 alike) : Product  RndMeth=Zero
  Sum : Sum
  Sum1 : Sum  Inputs=-+
  Trigonometric Function : Trigonometry  Operator=cos
  Trigonometric Function1 : Trigonometry
  d : Outport
  q : Outport  Port=2
  wires:
  [cos] -> Product/1
  alpha/1 -> Product/2, Product2/2
  Product/1 -> Sum/1
  Product1/1 -> Sum/2
  [sin] -> Product1/1
  beta/1 -> Product1/2, Product3/2
  [sin] -> Product2/1
  Product2/1 -> Sum1/1
  Product3/1 -> Sum1/2
  [cos] -> Product3/1
  Sum/1 -> d/1
  Sum1/1 -> q/1
  Trigonometric Function1/1 -> [sin]
  Trigonometric Function/1 -> [cos]
  wt/1 -> Trigonometric Function/1, Trigonometric Function1/1

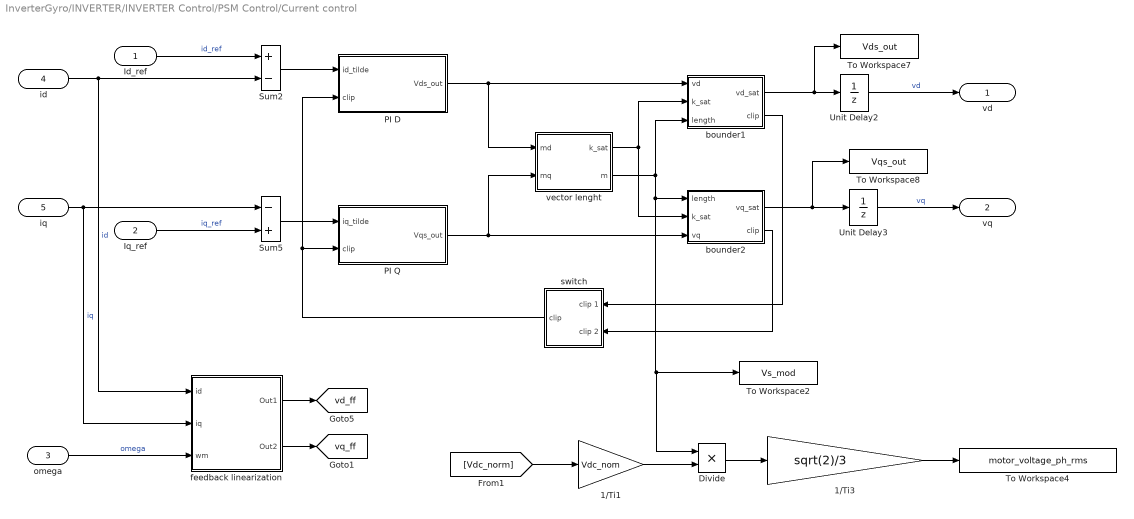
== system InverterGyro/INVERTER/INVERTER Control/PSM Control/Current control ==
  Id_ref : Inport
  Iq_ref : Inport  Port=2
  omega : Inport  Port=3
  id : Inport  Port=4
  iq : Inport  Port=5
  1/Ti1 : Gain  Gain=Vdc_nom  SaturateOnIntegerOverflow=on  OutDataTypeStr=Inherit: Same as input  ParamDataTypeStr=Inherit: Same as input
  1/Ti3 : Gain  Gain=sqrt(2)/3  SaturateOnIntegerOverflow=on  OutDataTypeStr=Inherit: Same as input  ParamDataTypeStr=Inherit: Same as input
  Divide : Product
  PI D : Subsystem
  PI Q : Subsystem
  Sum2 : Sum  Inputs=+-  SaturateOnIntegerOverflow=on
  Sum5 : Sum  Inputs=-+  SaturateOnIntegerOverflow=on
  To Workspace2 : ToWorkspace  VariableName=Vs_mod  SampleTime=Tsamp
      settings: MaxDataPoints=Nc
  To Workspace4 : ToWorkspace  VariableName=motor_voltage_ph_rms  SampleTime=Tsamp
      settings: MaxDataPoints=Nc
  To Workspace7 : ToWorkspace  VariableName=Vds_out  SampleTime=Tsamp
      settings: MaxDataPoints=Nc
  To Workspace8 : ToWorkspace  VariableName=Vqs_out  SampleTime=Tsamp
      settings: MaxDataPoints=Nc
  Unit Delay2 : UnitDelay  SampleTime=Tcontrol_INV  HasFrameUpgradeWarning=on
  Unit Delay3 : UnitDelay  SampleTime=Tcontrol_INV  HasFrameUpgradeWarning=on
  bounder1 : Subsystem
  bounder2 : Subsystem
  feedback linearization : Subsystem
  switch : Subsystem
  vector lenght : Subsystem
  vd : Outport
  vq : Outport  Port=2
  tag scope: vd_ff=global, vq_ff=global
  wires:
  Iq_ref/1 -> Sum5/2  "iq_ref"
  Unit Delay3/1 -> vq/1  "vq"
  Unit Delay2/1 -> vd/1  "vd"
  Id_ref/1 -> Sum2/1  "id_ref"
  vector lenght/1(k_sat) -> bounder1/2(k_sat), bounder2/2(k_sat)
  vector lenght/2(m) -> bounder1/3(length), bounder2/1(length), Divide/1, To Workspace2/1
  bounder1/1(vd_sat) -> Unit Delay2/1, To Workspace7/1
  bounder2/1(vq_sat) -> Unit Delay3/1, To Workspace8/1
  omega/1 -> feedback linearization/3(wm)  "omega"
  PI Q/1(Vqs_out) -> bounder2/3(vq), vector lenght/2(mq)
  Sum5/1 -> PI Q/1(iq_tilde)
  PI D/1(Vds_out) -> vector lenght/1(md), bounder1/1(vd)
  Sum2/1 -> PI D/1(id_tilde)
  switch/1(clip) -> PI Q/2(clip), PI D/2(clip)
  bounder1/2(clip) -> switch/1(clip 1)
  bounder2/2(clip) -> switch/2(clip 2)
  iq/1 -> Sum5/1, feedback linearization/2(iq)  "iq"
  id/1 -> feedback linearization/1(id), Sum2/2  "id"
  [Vdc_norm] -> 1/Ti1/1
  1/Ti1/1 -> Divide/2
  Divide/1 -> 1/Ti3/1
  1/Ti3/1 -> To Workspace4/1
  feedback linearization/1(Out1) -> [vd_ff]
  feedback linearization/2(Out2) -> [vq_ff]

== system InverterGyro/INVERTER/INVERTER Control/PSM Control/References ==
  note: d-Current-Reference (Field-weakening)
  note: q-Current-Reference
  Constant1 : Constant  Value=0
  FW : Subsystem
  MTPA : Subsystem
  MinMax : MinMax  Inputs=3
  To Workspace1 : ToWorkspace  VariableName=id_ref  SampleTime=Tsamp
      settings: MaxDataPoints=Nc
  To Workspace2 : ToWorkspace  VariableName=id_ref_fw  SampleTime=Tsamp
      settings: MaxDataPoints=Nc
  To Workspace3 : ToWorkspace  VariableName=id_ref_mtpa  SampleTime=Tsamp
      settings: MaxDataPoints=Nc
  To Workspace7 : ToWorkspace  VariableName=iq_ref  SampleTime=Tsamp
      settings: MaxDataPoints=Nc
  Id_ref : Outport
  Iq_ref : Outport  Port=2
  tag scope: id_ref=global, iq_ref=global
  wires:
  FW/1(Id_ref_fw) -> To Workspace2/1
  MTPA/1(Id_ref_mtpa) -> MinMax/1, To Workspace3/1
  MinMax/1 -> [id_ref], To Workspace1/1, Id_ref/1  "id_ref"
  Constant1/1 -> MinMax/2
  [T_ref] -> To Workspace7/1, [iq_ref], Iq_ref/1  "iq_ref"

== system InverterGyro/INVERTER/INVERTER Control/PSM Control/Speed control ==
  Rotor speed : Inport
  Speed ref : Inport  Port=2
  1/Ti : Gain  Gain=kp_w  SaturateOnIntegerOverflow=on  OutDataTypeStr=Inherit: Same as input  ParamDataTypeStr=Inherit: Same as input
  Sum : Sum  Inputs=|++
  Sum1 : Sum  Inputs=+++  SaturateOnIntegerOverflow=on
  Sum2 : Sum  Inputs=-+  SaturateOnIntegerOverflow=on
  Sum3 : Sum  Inputs=-+  SaturateOnIntegerOverflow=on
  To Workspace7 : ToWorkspace  VariableName=w_tilde  SampleTime=Tsamp
      settings: MaxDataPoints=Nc
  Unit Delay4 : UnitDelay  SampleTime=Tcontrol_INV  HasFrameUpgradeWarning=on
  iq_lim : Saturate  UpperLimit=iq_lim  LowerLimit=-iq_lim
  kp : Gain  Gain=ki_w*Tcontrol_INV  SaturateOnIntegerOverflow=on  OutDataTypeStr=Inherit: Same as input  ParamDataTypeStr=Inherit: Same as input
  Torque ref : Outport
  wires:
  1/Ti/1 -> Sum1/1, Sum3/1
  kp/1 -> Sum1/2
  Sum2/1 -> To Workspace7/1, kp/1, 1/Ti/1
  Sum3/1 -> Unit Delay4/1
  Unit Delay4/1 -> Sum1/3
  Speed ref/1 -> Sum2/2
  Rotor speed/1 -> Sum2/1
  Sum1/1 -> iq_lim/1
  Sum/1 -> Torque ref/1
  iq_lim/1 -> Sum3/2, Sum/1

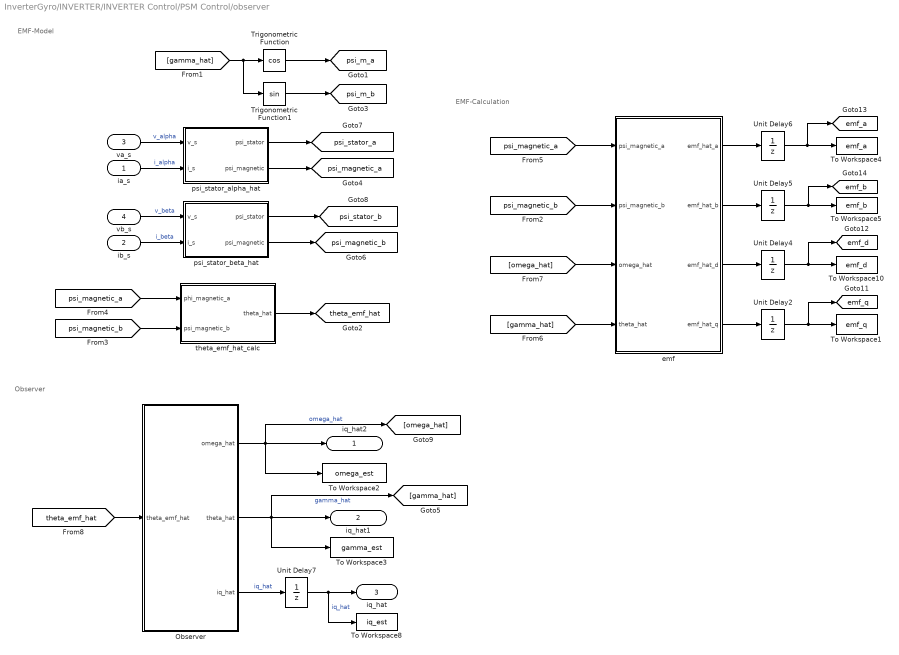
== system InverterGyro/INVERTER/INVERTER Control/PSM Control/observer ==
  note: EMF-Calculation
  note: EMF-Model
  note: Observer
  ia_s : Inport
  ib_s : Inport  Port=2
  va_s : Inport  Port=3
  vb_s : Inport  Port=4
  Observer : Subsystem
  To Workspace1 : ToWorkspace  VariableName=emf_q  SampleTime=Tsamp
      settings: MaxDataPoints=Nc
  To Workspace10 : ToWorkspace  VariableName=emf_d  SampleTime=Tsamp
      settings: MaxDataPoints=Nc
  To Workspace2 : ToWorkspace  VariableName=omega_est  SampleTime=Tsamp
      settings: MaxDataPoints=Nc
  To Workspace3 : ToWorkspace  VariableName=gamma_est  SampleTime=Tsamp
      settings: MaxDataPoints=Nc
  To Workspace4 : ToWorkspace  VariableName=emf_a  SampleTime=Tsamp
      settings: MaxDataPoints=Nc
  To Workspace5 : ToWorkspace  VariableName=emf_b  SampleTime=Tsamp
      settings: MaxDataPoints=Nc
  To Workspace8 : ToWorkspace  VariableName=iq_est  SampleTime=Tsamp
      settings: MaxDataPoints=Nc
  Trigonometric Function : Trigonometry  Operator=cos
  Trigonometric Function1 : Trigonometry
  Unit Delay{2,4..7} (5 alike) : UnitDelay  SampleTime=Tcontrol_INV  HasFrameUpgradeWarning=on
  emf : Subsystem
  psi_stator_alpha_hat : Subsystem
  psi_stator_beta_hat : Subsystem
  theta_emf_hat_calc : Subsystem
  iq_hat2 : Outport
  iq_hat1 : Outport  Port=2
  iq_hat : Outport  Port=3
  tag scope: emf_a=global, emf_b=global, emf_d=global, emf_q=global, psi_m_a=global, psi_m_b=global, psi_magnetic_a=global, psi_magnetic_b=global, psi_stator_a=global, psi_stator_b=global, theta_emf_hat=global
  wires:
  Trigonometric Function/1 -> [psi_m_a]
  Trigonometric Function1/1 -> [psi_m_b]
  ia_s/1 -> psi_stator_alpha_hat/2(i_s)  "i_alpha"
  psi_stator_alpha_hat/1(psi_stator) -> [psi_stator_a]
  ib_s/1 -> psi_stator_beta_hat/2(i_s)  "i_beta"
  psi_stator_beta_hat/1(psi_stator) -> [psi_stator_b]
  psi_stator_alpha_hat/2(psi_magnetic) -> [psi_magnetic_a]
  psi_stator_beta_hat/2(psi_magnetic) -> [psi_magnetic_b]
  [psi_magnetic_a] -> theta_emf_hat_calc/1(phi_magnetic_a)
  [psi_magnetic_b] -> theta_emf_hat_calc/2(psi_magnetic_b)
  theta_emf_hat_calc/1(theta_hat) -> [theta_emf_hat]
  [psi_magnetic_b] -> emf/2(psi_magnetic_b)
  [psi_magnetic_a] -> emf/1(psi_magnetic_a)
  [gamma_hat] -> emf/4(theta_hat)
  [omega_hat] -> emf/3(omega_hat)
  emf/1(emf_hat_a) -> Unit Delay6/1
  [theta_emf_hat] -> Observer/1(theta_emf_hat)
  Observer/2(theta_hat) -> To Workspace3/1, [gamma_hat], iq_hat1/1  "gamma_hat"
  Observer/1(omega_hat) -> [omega_hat], To Workspace2/1, iq_hat2/1  "omega_hat"
  va_s/1 -> psi_stator_alpha_hat/1(v_s)  "v_alpha"
  vb_s/1 -> psi_stator_beta_hat/1(v_s)  "v_beta"
  Unit Delay4/1 -> [emf_d], To Workspace10/1
  Unit Delay2/1 -> [emf_q], To Workspace1/1
  Unit Delay6/1 -> To Workspace4/1, [emf_a]
  Unit Delay5/1 -> To Workspace5/1, [emf_b]
  emf/2(emf_hat_b) -> Unit Delay5/1
  emf/3(emf_hat_d) -> Unit Delay4/1
  emf/4(emf_hat_q) -> Unit Delay2/1
  [gamma_hat] -> Trigonometric Function1/1, Trigonometric Function/1
  Unit Delay7/1 -> iq_hat/1, To Workspace8/1  "iq_hat"
  Observer/3(iq_hat) -> Unit Delay7/1  "iq_hat"

== system InverterGyro/INVERTER/INVERTER Control/PSM Control/speed reference ==
  1/Ti2 : Gain  Gain=sign_speed/Omega_bez_plant_m  SaturateOnIntegerOverflow=on  OutDataTypeStr=Inherit: Same as input  ParamDataTypeStr=Inherit: Same as input
  1/Ti3 : Gain  Gain=wref^2/3  SaturateOnIntegerOverflow=on  OutDataTypeStr=Inherit: Same as input  ParamDataTypeStr=Inherit: Same as input
  Rate Limiter : RateLimiter  RisingSlewLimit=wref/6  FallingSlewLimit=-wref/6  SampleTimeMode=inherited
  Saturation : Saturate  UpperLimit=wref  LowerLimit=0
  Saturation1 : Saturate  UpperLimit=wref  LowerLimit=-wref
  Sum : Sum  Inputs=|+-
  Zero-Order Hold8 : ZeroOrderHold  SampleTime=Tcontrol_INV
  wref : simulink/Sources/Ramp  slope=2*wref/tref  start=start_torque_control  InitialOutput=0
  ref_out : Outport
  tag scope: omega_ref=global
  wires:
  Zero-Order Hold8/1 -> 1/Ti2/1
  wref/1 -> Saturation/1
  Saturation/1 -> Sum/1
  Sum/1 -> Zero-Order Hold8/1
  1/Ti2/1 -> [omega_ref], ref_out/1
  Saturation1/1 -> Sum/2
  1/Ti3/1 -> Rate Limiter/1
  Rate Limiter/1 -> Saturation1/1
  [force_ramp_down] -> 1/Ti3/1

== system InverterGyro/INVERTER/INVERTER Control/abc2dq /abc2alphabeta ==
  a : Inport
  b : Inport  Port=2
  c : Inport  Port=3
  Gain1 : Gain  Gain=-1/2
  Gain11 : Gain  Gain=-1/2
  Gain2 : Gain  Gain=0
  Gain3 : Gain  Gain=sqrt(3)/2
  Gain4 : Gain  Gain=-sqrt(3)/2
  Gain8 : Gain  Gain=2/3
  Gain9 : Gain  Gain=2/3
  Sum : Sum  Inputs=+++
  Sum1 : Sum  Inputs=+++
  "alpha " : Outport
  "beta " : Outport  Port=2
  wires:
  Sum1/1 -> Gain9/1
  Sum/1 -> Gain8/1
  b/1 -> Gain11/1, Gain3/1
  c/1 -> Gain1/1, Gain4/1
  a/1 -> Sum/1, Gain2/1
  Gain4/1 -> Sum1/3
  Gain3/1 -> Sum1/2
  Gain2/1 -> Sum1/1
  Gain1/1 -> Sum/3
  Gain11/1 -> Sum/2
  Gain8/1 -> "alpha "/1
  Gain9/1 -> "beta "/1

== system InverterGyro/INVERTER/INVERTER Control/abc2dq /alphabeta2dq ==
  note: va=V cos(wt)
      | vb=V cos(wt-2pi/3)
      | vc=V cos(wt+2pi/3)
  alpha : Inport
  beta : Inport  Port=2
  wt : Inport  Port=3
  Gain : Gain
  Gain1 : Gain
  Product{,1..3} (4 alike) : Product  RndMeth=Zero
  Sum : Sum
  Sum1 : Sum  Inputs=-+
  Trigonometric Function : Trigonometry  Operator=cos
  Trigonometric Function1 : Trigonometry
  d : Outport
  q : Outport  Port=2
  wires:
  wt/1 -> Trigonometric Function1/1, Trigonometric Function/1
  Trigonometric Function/1 -> [cos]
  Trigonometric Function1/1 -> [sin]
  Gain1/1 -> q/1
  Gain/1 -> d/1
  Sum1/1 -> Gain1/1
  [cos] -> Product3/1
  Product3/1 -> Sum1/2
  Product2/1 -> Sum1/1
  [sin] -> Product2/1
  Sum/1 -> Gain/1
  beta/1 -> Product3/2, Product1/2
  [sin] -> Product1/1
  Product1/1 -> Sum/2
  Product/1 -> Sum/1
  alpha/1 -> Product2/2, Product/2
  [cos] -> Product/1

== system InverterGyro/INVERTER/INVERTER Control/cabcd/latch ==
  in : Inport
  en : Inport  Port=2
  Constant2 : Constant  Value=0
  D Flip-Flop : simulink_extras/Flip Flops/D Flip-Flop
  Data Type Conversion : DataTypeConversion  OutDataTypeStr=double
  Data Type Conversion1 : DataTypeConversion  OutDataTypeStr=boolean
  Logical Operator : Logic  Operator=NOT  AllPortsSameDT=off  OutDataTypeStr=boolean
  S-R Flip-Flop : simulink_extras/Flip Flops/S-R Flip-Flop  initial_condition=0
  Sum : Sum  Inputs=|++
  Switch2 : Switch  Threshold=0.5
  Unit Delay : UnitDelay  SampleTime=Tcontrol_INV  HasFrameUpgradeWarning=on
  out : Outport
  wires:
  en/1 -> Switch2/2
  in/1 -> Switch2/1
  Constant2/1 -> Switch2/3
  Switch2/1 -> Data Type Conversion1/1
  D Flip-Flop/2 -> Unit Delay/1, Data Type Conversion/1
  Logical Operator/1 -> D Flip-Flop/2
  Data Type Conversion1/1 -> D Flip-Flop/1, Logical Operator/1
  Unit Delay/1 -> S-R Flip-Flop/1
  S-R Flip-Flop/1 -> D Flip-Flop/3
  [enable_RGM_module] -> Sum/2
  Data Type Conversion/1 -> Sum/1
  Sum/1 -> out/1

== system InverterGyro/INVERTER/INVERTER Control/cabcd/latch  ==
  in : Inport
  en : Inport  Port=2
  Constant2 : Constant  Value=0
  D Flip-Flop : simulink_extras/Flip Flops/D Flip-Flop
  Data Type Conversion : DataTypeConversion  OutDataTypeStr=double
  Data Type Conversion1 : DataTypeConversion  OutDataTypeStr=boolean
  Logical Operator : Logic  Operator=NOT  AllPortsSameDT=off  OutDataTypeStr=boolean
  S-R Flip-Flop : simulink_extras/Flip Flops/S-R Flip-Flop  initial_condition=0
  Switch2 : Switch  Threshold=0.5
  Unit Delay : UnitDelay  SampleTime=Tcontrol_INV  HasFrameUpgradeWarning=on
  out : Outport
  wires:
  S-R Flip-Flop/1 -> D Flip-Flop/3
  Unit Delay/1 -> S-R Flip-Flop/1
  Data Type Conversion1/1 -> Logical Operator/1, D Flip-Flop/1
  Logical Operator/1 -> D Flip-Flop/2
  D Flip-Flop/2 -> Unit Delay/1
  Switch2/1 -> Data Type Conversion1/1
  Constant2/1 -> Switch2/3
  in/1 -> Switch2/1
  en/1 -> Switch2/2
  Data Type Conversion/1 -> out/1
  D Flip-Flop/1 -> Data Type Conversion/1

== system InverterGyro/INVERTER/INVERTER Control/dq2alphabeta2/dq-alphabeta ==
  note: va=V cos(wt)
      | vb=V cos(wt-2pi/3)
      | vc=V cos(wt+2pi/3)
  d : Inport
  q : Inport  Port=2
  wt : Inport  Port=3
  Product{,1..3} (4 alike) : Product  RndMeth=Zero
  Sum : Sum  Inputs=+-
  Sum1 : Sum
  Trigonometric Function : Trigonometry  Operator=cos
  Trigonometric Function1 : Trigonometry
  alpha : Outport
  beta : Outport  Port=2
  wires:
  Sum1/1 -> beta/1
  [cos] -> Product3/1
  Product3/1 -> Sum1/2
  Product2/1 -> Sum1/1
  [sin] -> Product2/1
  Sum/1 -> alpha/1
  q/1 -> Product3/2, Product1/2
  [sin] -> Product1/1
  Product1/1 -> Sum/2
  Product/1 -> Sum/1
  d/1 -> Product2/2, Product/2
  [cos] -> Product/1
  Trigonometric Function1/1 -> [sin]
  Trigonometric Function/1 -> [cos]
  wt/1 -> Trigonometric Function/1, Trigonometric Function1/1
